simulink model "QD2_DroneStack_PID_AM32ESC_R2022b"  (R2022b)
settings: Solver=ode1  StartTime=0.0  StopTime=inf  FixedStep=1/1000  RelTol=1e-3  EnableMultiTasking=on
InitFcn:
  | Motor_Mapping_7_Inch
model workspace (MAT data in the model file):
  target_system = 1
undefined symbols (not defined in the file): _Commander, _QDrone2, _Stabilizer, datetime, HIL, KT, lf, log_, log_QD2_, m, Motor_Matrix, n, qc_get_step_size, s, saved_data
libraries: quarc_library x170, simulink x35, simulink_extras x11
(part 7 of 7)

== matlab function QD2_DroneStack_PID_AM32ESC_R2022b/QDrone 2 DAQ/MATLAB Function ==
  data: mdl_time input; arm input; estop input; esc_problem input; cmd output; cmd_enable output; tele_enable output; esc_ready output; esc_timeout output; stop_mdl output; pre_state input; state output
function [cmd, cmd_enable, tele_enable, esc_ready, esc_timeout, stop_mdl, state] = esc_state_machine(mdl_time, arm, estop, esc_problem, pre_state)

persistent next_state_after_pause
persistent state_counter
persistent state_counter_after_pause
persistent esc_timeout_state

% Define state enumeration
STATE_INIT_WAIT = 0;
STATE_INIT_WAIT_EXTENDED = 1;
STATE_IDLE = 2;
STATE_CMD_BEEP = 3;
STATE_CMD_SET_DIRECTION = 4;
STATE_CMD_MOTOR = 5;
STATE_CMD_ZERO = 77;
STATE_CMD_DISABLED = 88;
STATE_EXIT = 99;

% Define state counter values
COUNT_STATE_INIT_MIN = 1000;
COUNT_STATE_INIT_MAX = 10000;
COUNT_STATE_IDLE = 1000;
COUNT_STATE_BEEP = 60;
%COUNT_STATE_BEEP = 1000;
COUNT_STATE_SET_DIRECTION = 120;
%COUNT_STATE_SET_DIRECTION = 500;
COUNT_STATE_DISABLE_BEEP = 1000;
COUNT_STATE_DISABLE_DIRECTION = 500;
COUNT_STATE_CMD_ZERO_PAUSE = 1000;


% Initialize persistent variables
if isempty(next_state_after_pause)
    next_state_after_pause = STATE_EXIT;
end
if isempty(state_counter)
    state_counter=COUNT_STATE_INIT_MIN;
end
if isempty(state_counter_after_pause)
    state_counter_after_pause = COUNT_STATE_IDLE;
end
if isempty(esc_timeout_state)
    esc_timeout_state = 0;
end


% Initialize output
state = STATE_INIT_WAIT;
cmd = [0,0,0,0];
tele_enable = 0;
cmd_enable = 0;
stop_mdl = 0;
esc_ready = 0;

% State Transition
% E-Stop superceeds all commands
if estop
    state = STATE_EXIT;
else
    switch pre_state
        % Initialization - send command zero and request telemetry
        case STATE_INIT_WAIT
            state_counter = state_counter - 1;
            if state_counter <= 0 
                % Go to next state
                state = STATE_INIT_WAIT_EXTENDED;
                state_counter = COUNT_STATE_INIT_MAX;
            else
                % Stay in current state
                state = pre_state;
            end
    
    
        % Extended initialization wait until ESC initialization completed
        case STATE_INIT_WAIT_EXTENDED
            state_counter = state_counter - 1;
            if state_counter <= 0
                % Max timeout reached, unrecoverable error condition, flag and
                % terminate.
                state = STATE_EXIT;
                esc_timeout_state = 1;
                
            else
                % Check if we are clear to proceed
                if esc_problem
                    % Stay in current state and keep waiting
                    state = pre_state;
                else
                    % Go to next state
                    state = STATE_CMD_ZERO;
                    state_counter = COUNT_STATE_CMD_ZERO_PAUSE;
                    next_state_after_pause = STATE_CMD_BEEP;
                    state_counter_after_pause = COUNT_STATE_BEEP;
                end
            end
    
        % Send Beep command
        case STATE_CMD_BEEP
            state_counter = state_counter - 1;
            if state_counter <= 0
                % Go to next state
                state = STATE_CMD_DISABLED;
                state_counter = COUNT_STATE_DISABLE_BEEP;
                next_state_after_pause = STATE_CMD_SET_DIRECTION;
                state_counter_after_pause = COUNT_STATE_SET_DIRECTION;
                % Alternately go directly to set direction
%                 state = STATE_CMD_SET_DIRECTION;
%                 state_counter = COUNT_STATE_SET_DIRECTION;
            else
                % Stay in current state
                state = pre_state;
            end
            
        % Set Direction
        case STATE_CMD_SET_DIRECTION
            state_counter = state_counter - 1;
            if state_counter <= 0
                % Go to next state
                state = STATE_CMD_DISABLED;
                state_counter = COUNT_STATE_DISABLE_DIRECTION;
                next_state_after_pause = STATE_IDLE;
                state_counter_after_pause = COUNT_STATE_IDLE;
            else
                % Stay in current state
                state = pre_state;
            end
    
        % Idle/Disarm state with telemetry enabled
        case STATE_IDLE
            if arm
                % Go to next state
                state = STATE_CMD_MOTOR;
            else
                % Stay and wait
                state = pre_state;
            end
            
        % Drive motor
        case STATE_CMD_MOTOR
            % Skip checking for telemetry fails after motor starts
%            if not(esc_problem)
                if not(arm)
                    % Go to next state
                    state = STATE_IDLE;
                else
                    % Stay in current state
                    state = pre_state;
                end
%             else
%                 % Not expecting this but flag it
%                 state = STATE_EXIT;
%                 esc_timeout_state = 1;
%             end
    
        % Pause with command disabled
        case STATE_CMD_DISABLED
            state_counter = state_counter - 1;
            if state_counter <= 0
                % Go to next state
                state = next_state_after_pause;
                state_counter = state_counter_after_pause;
            else
                % stay in current state
                state = pre_state;
            end
            
        % Generic pause state with command and telemetry enabled
        case STATE_CMD_ZERO
            state_counter = state_counter - 1;
            if state_counter <= 0
                % Got to next state
                state = next_state_after_pause;
                state_counter = state_counter_after_pause;
            else
                % Stay in current state
                state = pre_state;
            end 

        % Exit state
        case STATE_EXIT
            % Do nothing until model stop
            state = pre_state;
    end
end

% State Output
switch state
    % Command zero to initialize the ESC
    case STATE_INIT_WAIT
        cmd = [0, 0, 0, 0];
        tele_enable = 1;
        cmd_enable = 1;
        stop_mdl = 0;
        esc_ready = 0;

    % Extended wait during initialization to confirm all ESC are ready
    case STATE_INIT_WAIT_EXTENDED
        cmd = [0,0,0,0];
        tele_enable = 1;
        cmd_enable = 1;
        stop_mdl = 0;
        esc_ready = 0;

    % Send beep command
    case STATE_CMD_BEEP
        cmd = [1, 1, 1, 1]*3;
        %tele_enable = 0;
        % Old BLHeli firmware needs the telemetry bit set to accept beep
        % command
        tele_enable = 1;
        cmd_enable = 1;
        stop_mdl = 0;
        esc_ready = 0;

    % Set Direction
    case STATE_CMD_SET_DIRECTION
        % Normal - for old BLHeli firmware
        cmd = [20, 21, 21, 20];
        % Workaround - for new AM32 firmware - looks like a bug  
        %cmd = [21, 20, 20, 21];
        %cmd = [21, 21, 21, 21];
        %cmd = [20, 20, 20, 20];
        %tele_enable = 0;
        % old BLHeli firmware needs the telemetry bit set to accept set
        % direction command
        tele_enable = 1;
        cmd_enable = 1;
        stop_mdl = 0;
        esc_ready = 0;

    % Disarm command
    case STATE_IDLE
        cmd = [0,0,0,0];
        tele_enable = 0;
        cmd_enable = 1;
        stop_mdl = 0;
        esc_ready = 1;
        
    % Drive motors
    case STATE_CMD_MOTOR
        cmd = [48, 48, 48, 48];
        tele_enable = 1;
        cmd_enable = 1;
        stop_mdl = 0;
        esc_ready = 1;

    % Idle/disable state
    case STATE_CMD_DISABLED
        cmd = [0 0 0 0];
        tele_enable = 0;
        cmd_enable = 0;
        stop_mdl = 0;
        esc_ready = 0;

    % Generic Pause
    case STATE_CMD_ZERO
        cmd = [0,0,0,0];
        tele_enable = 1;
        cmd_enable = 1;
        stop_mdl = 0;
        esc_ready = 0;

    % Stop
    case STATE_EXIT
        cmd = [0,0,0,0];
        tele_enable = 0;
        cmd_enable = 1;
        stop_mdl = 1;
        esc_ready = 0;
end

% output esc_timeout variable
esc_timeout = esc_timeout_state;

== matlab function QD2_DroneStack_PID_AM32ESC_R2022b/QDrone 2 DAQ/Force to percentage Mapping ==
  data: V_Bat_Act input; Motor_Forces input; Duty_Cycle output; KT input
function Duty_Cycle = fcn(V_Bat_Act,Motor_Forces,KT)

B = KT(2)^2-4*KT(1)*(KT(3)-Motor_Forces)

invalid_signal = B < 0
B(invalid_signal) = 0

% Ranges from 1000-2000
Volt_CMD_Theo = -0.5*KT(2)/KT(1)+ sqrt(B)/(2*KT(1));

Duty_Cycle = Volt_CMD_Theo/V_Bat_Act;

== matlab function QD2_DroneStack_PID_AM32ESC_R2022b/QDrone2 DAQ - Outdated/Attitude Estimate from IMU Data/For Each Subsystem - Attitutde Estimates/roll and pitch approximation from accelerometer ==
  data: roll_acc output; pitch_acc output; acc_body input
function [roll_acc, pitch_acc]   = fcn(acc_body)
%#eml
n = norm(acc_body,2);
if n>eps
    acc_body = acc_body/n; 
else
    acc_body = [0 0 1]';
end

roll_acc = atan2(acc_body(2),acc_body(3));
pitch_acc = atan2( -acc_body(1), acc_body(2)*sin(roll_acc)+acc_body(3)*cos(roll_acc));

== matlab function QD2_DroneStack_PID_AM32ESC_R2022b/QDrone2 DAQ - Outdated/Subsystem/MATLAB Function LED Color Assignment ==
  data: E_Stop input; Arm input; value output; low_battery input
function value = fcn(E_Stop, Arm, low_battery)

if low_battery == 1|| E_Stop ==1
    value = 1;
elseif Arm == 1 & E_Stop ==0
    value = 2;
elseif Arm == 0 && E_Stop == 0 
    value = 3;
else 
    value = 3;
end

== matlab function QD2_DroneStack_PID_AM32ESC_R2022b/COMMANDER (ANGLE MODE)/THROTTLE SWITCHBOX /Throttle Switchbox ==
  data: FSM_state input; sigmoid output
function sigmoid  = application_drone_throttle_switchbox(FSM_state)

% Application Drone: Throttle Switchbox
%
% Logic for switching between throttle commands from the controller 
%
% v2.0 - 5th october, 2018
%
% INPUTS:
% -------
% FSM_state = current state of the FSM------------------------------------------------------- (#)         [1]
% 
% OUTPUTS:
% --------
% sigmoid = an integer whose state determines how the heights are transformed---------------- (#)         [1]
% sigmoid = 1 - Command 0 throttle
% sigmoid = 2 - Sigmoid throttle up from 0 to the trim value
% sigmoid = 3 - Pass controller throttle straight through + trim value.
% sigmoid = 4 - Ignore controller throttle. Sigmoid it down to 0.
% sigmoid = 5 - Pass controller throttle straight through + trim value.


sigmoid = 0;
switch FSM_state
    case 1 % IDLE STATE
        sigmoid = 1;
    case 2 % ARM STATE
        sigmoid = 1;
    case 3 % TAKEOFF THROTTLE STATE
        sigmoid = 2;
    case 4 % TAKEOFF HEIGHT STATE
        sigmoid = 3;
    case 5 % FLIGHT STATE
        sigmoid = 3;
    case 6 % AUTOLAND STATE
        sigmoid = 5;
    case 7 % EMERGENCY STOP STATE
        sigmoid = 4;
    case 8 % EMERGENCY ABORT STATE
        sigmoid = 1;
    case 9 % DISABLE STATE
        sigmoid = 1;
end

== matlab function QD2_DroneStack_PID_AM32ESC_R2022b/QDrone2 DAQ - Outdated/MotorCMD_FSM ==
  data: Arm_Signal input; E_Stop input; ESC_cmd output; Motor_State output; Model_Time input; Motor_State input
function [ESC_cmd,Motor_State]= fcn(Arm_Signal,E_Stop,Model_Time, Motor_State)

persistent state ESC_CMD 

%  Initialize motor state at the start of the model
if isempty(state)
    state = 2;
    ESC_CMD = zeros(1,4);
end 

% ESC Numbers w.r.t motor positions on QDrone: 
%         FRONT
%       4(3)       2(1)
% 
%       3(2)       1(0)
%          BACK  


% ============ Motor programing state machine ============ 

% State machine transitions: 

% Motor configuration state: 
if E_Stop == 0 && state ~= 9
    % Start with the motors in an idle state    
    if state == 2 && Model_Time > 0 && Model_Time <= 1  
        if Arm_Signal == 1
            % Error state, you started the model while the QDrone was armed
            state = 9;
        end 
           
    elseif state ==2  && Model_Time > 1 && Model_Time <= 2
        % Enter motor Low Frequency state:
        state = 1;
        
    elseif state ==1  && Model_Time > 2 && Model_Time <= 2.5
        % Set motor orientation
        state = 0;
        
    elseif state == 0 && Model_Time > 2.5    
        % Enter motor idle state: 
        state = 2; 

    elseif Motor_State ==2 && Arm_Signal == 1 
        % Enter arm state 
        state = 3;

    elseif Motor_State ==3 && Arm_Signal ==0 
        % Return to idle state 
        state = 2; 
    end 
    
elseif E_Stop ==1 
    % You've entered emergency state, disarm QDrone2!
    state = 9; 
end 


% State Machine commands: 
switch state 
    
    % ESC orientation set:
    case 0
        % for all drones
        ESC_CMD = [20,21,21,20];
        %for 1st R&D Drone 
        % ESC_CMD = [0,0,0,0];
    
    % Motor Low Frequency Beep:
    case 1
        ESC_CMD = [1,1,1,1];
    
    % Enter motor stop state: 
    case 2
        ESC_CMD = [0,0,0,0];
    
    % Motors in Arm State:
    case 3
        ESC_CMD = [48,48,48,48];
        
    % Same as state 2 but used as an Error State to stop motor cmd:
    case 9
        ESC_CMD = [0,0,0,0];
        
end 
    


Motor_State = state;
ESC_cmd = ESC_CMD;

Motor_State, ESC_cmd;

== matlab function QD2_DroneStack_PID_AM32ESC_R2022b/HORIZON FRAME CONVERSION AND ESTIMATION/Pose Switchbox/MATLAB Function ==
  data: sigmoid_type input; enable output; x_des input; slow_lim input; fast_lim input; x_cur input; x_vel input; x_ref output; max_x_vel output; max_x_accel output; x_meas input
function [enable, x_ref, max_x_vel, max_x_accel] = fcn(sigmoid_type, x_des, slow_lim, fast_lim, x_cur, x_vel, x_meas)

% Note: Some of the cases below are identical. However, they are separated out 
% based on the states of the state machine for ease of modification in the future. 
% For example, states 4 and 5 are identical. However, if the user wants different 
% signmoid behaviour when taking off than when landing, these cases may not be the same. 

enable = 0;
x_ref = 0;
max_x_vel = 0;
max_x_accel = 0;

switch sigmoid_type
    case 1 % This is for the IDLE, ARM, E_ABORT, E_STOP and DISABLE states of the FSM
        enable = 1;
        x_ref = x_meas;
        max_x_vel = slow_lim(1);
        max_x_accel = slow_lim(2);

    case 2 % This is for the TAKEOFF THROTTLE state of the FSM
        enable = 1;
        x_ref = x_meas;
        max_x_vel = slow_lim(1);
        max_x_accel = slow_lim(2);

    case 3 % This is for the FLIGHT state of the FSM
        enable = 1;
        x_ref = x_des;
        max_x_vel = fast_lim(1);
        max_x_accel = fast_lim(2);

    case 4 % This is for the TAKEOFF HEIGHT state of the FSM
        enable = 1;
        x_ref = x_des;
        if (abs(x_cur - x_des) <= 0.02)
            max_x_vel = fast_lim(1);
            max_x_accel = fast_lim(2);
        else    
            max_x_vel = slow_lim(1);
            max_x_accel = slow_lim(2);
        end
    case 5 % This is for the AUTOLAND state of the FSM
        enable = 1;
        x_ref = x_des;
        if (abs(x_cur - x_des) <= 0.02)
            max_x_vel = fast_lim(1);
            max_x_accel = fast_lim(2);        
        else
            max_x_vel = slow_lim(1);
            max_x_accel = slow_lim(2);
        end
        
end

== matlab function QD2_DroneStack_PID_AM32ESC_R2022b/HORIZON FRAME CONVERSION AND ESTIMATION/Pose Switchbox/MATLAB Function1 ==
  data: sigmoid_type input; enable output; y_des input; slow_lim input; fast_lim input; y_cur input; y_vel input; y_ref output; max_y_vel output; max_y_accel output; y_meas input
function [enable, y_ref, max_y_vel, max_y_accel] = fcn(sigmoid_type, y_des, slow_lim, fast_lim, y_cur, y_vel, y_meas)

% Note: Some of the cases below are identical. However, they are separated out 
% based on the states of the state machine for ease of modification in the future. 
% For example, states 4 and 5 are identical. However, if the user wants different 
% signmoid behaviour when taking off than when landing, these cases may not be the same. 

enable = 0;
y_ref = 0;
max_y_vel = 0;
max_y_accel = 0;

switch sigmoid_type
    case 1 % This is for the IDLE, ARM, E_ABORT, E_STOP and DISABLE states of the FSM
        enable = 1;
        y_ref = y_meas;
        max_y_vel = slow_lim(1);
        max_y_accel = slow_lim(2);

    case 2 % This is for the TAKEOFF THROTTLE state of the FSM
        enable = 1;
        y_ref = y_meas;
        max_y_vel = slow_lim(1);
        max_y_accel = slow_lim(2);

    case 3 % This is for the FLIGHT state of the FSM
        enable = 1;
        y_ref = y_des;
        max_y_vel = fast_lim(1);
        max_y_accel = fast_lim(2);

    case 4 % This is for the TAKEOFF HEIGHT state of the FSM
        enable = 1;
        y_ref = y_des;
        if (abs(y_cur - y_des) <= 0.02)
            max_y_vel = fast_lim(1);
            max_y_accel = fast_lim(2);
        else    
            max_y_vel = slow_lim(1);
            max_y_accel = slow_lim(2);
        end
    case 5 % This is for the AUTOLAND state of the FSM
        enable = 1;
        y_ref = y_des;
        if (abs(y_cur - y_des) <= 0.02)
            max_y_vel = fast_lim(1);
            max_y_accel = fast_lim(2);        
        else
            max_y_vel = slow_lim(1);
            max_y_accel = slow_lim(2);
        end
        
end
